simulink model "BMS_Protection_Logic"  (R2024a)
settings: Solver=VariableStepAuto  StartTime=0.0  StopTime=10.0  RelTol=1e-3
settings Model: Creator=gopin  LastModifiedBy=gopin

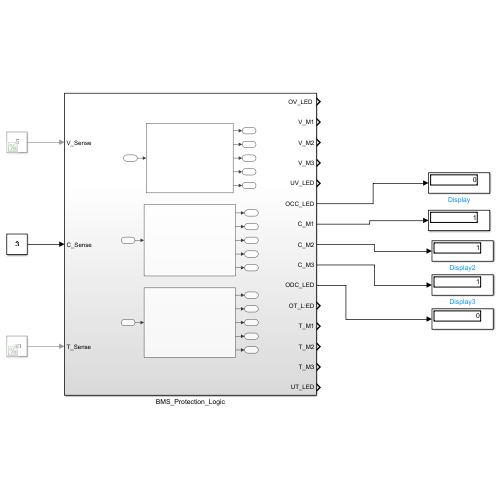
[thumbnail: Simulink's stored preview of the top-level diagram]
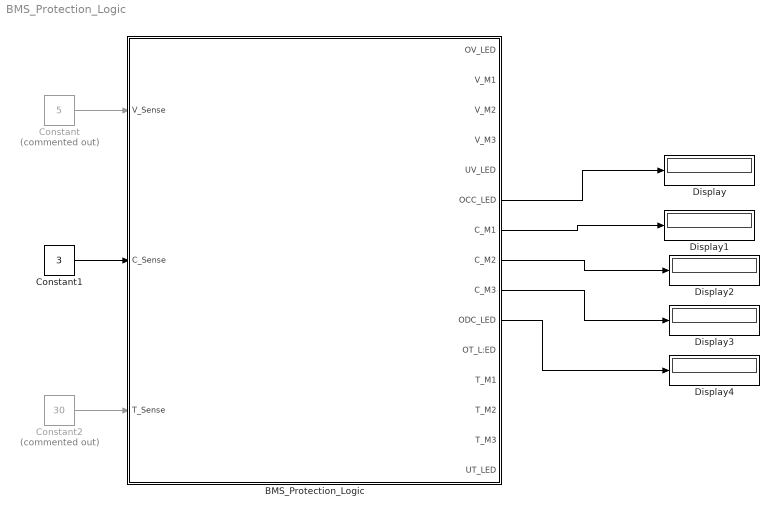
== system BMS_Protection_Logic ==
  BMS_Protection_Logic : Subsystem
  Constant : Constant  Commented=on  Value=5
  Constant1 : Constant  Value=3
  Constant2 : Constant  Commented=on  Value=30
  Display{,1..4} (5 alike) : Display
  wires:
  Constant/1 -> BMS_Protection_Logic/1(V_Sense)
  Constant1/1 -> BMS_Protection_Logic/2(C_Sense)
  Constant2/1 -> BMS_Protection_Logic/3(T_Sense)
  BMS_Protection_Logic/6(OCC_LED) -> Display/1
  BMS_Protection_Logic/7(C_M1) -> Display1/1
  BMS_Protection_Logic/8(C_M2) -> Display2/1
  BMS_Protection_Logic/9(C_M3) -> Display3/1
  BMS_Protection_Logic/10(ODC_LED) -> Display4/1

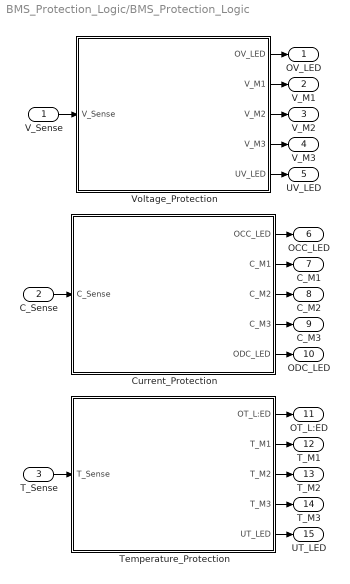
== system BMS_Protection_Logic/BMS_Protection_Logic ==
  V_Sense : Inport
  C_Sense : Inport  Port=2
  T_Sense : Inport  Port=3
  Current_Protection : Subsystem
  Temperature_Protection : Subsystem
  Voltage_Protection : Subsystem
  "OV_LED " : Outport
  V_M1 : Outport  Port=2
  V_M2 : Outport  Port=3
  V_M3 : Outport  Port=4
  UV_LED : Outport  Port=5
  OCC_LED : Outport  Port=6
  C_M1 : Outport  Port=7
  C_M2 : Outport  Port=8
  C_M3 : Outport  Port=9
  ODC_LED : Outport  Port=10
  OT_L:ED : Outport  Port=11
  T_M1 : Outport  Port=12
  T_M2 : Outport  Port=13
  T_M3 : Outport  Port=14
  UT_LED : Outport  Port=15
  wires:
  V_Sense/1 -> Voltage_Protection/1(V_Sense)
  Voltage_Protection/1("OV_LED ") -> "OV_LED "/1
  C_Sense/1 -> Current_Protection/1(C_Sense)
  Current_Protection/2(C_M1) -> C_M1/1
  Temperature_Protection/5(UT_LED) -> UT_LED/1
  Voltage_Protection/2(V_M1) -> V_M1/1
  Temperature_Protection/2(T_M1) -> T_M1/1
  Voltage_Protection/3(V_M2) -> V_M2/1
  Voltage_Protection/4(V_M3) -> V_M3/1
  Current_Protection/5(ODC_LED) -> ODC_LED/1
  Voltage_Protection/5(UV_LED) -> UV_LED/1
  Current_Protection/1(OCC_LED) -> OCC_LED/1
  Current_Protection/3(C_M2) -> C_M2/1
  Temperature_Protection/1(OT_L:ED) -> OT_L:ED/1
  T_Sense/1 -> Temperature_Protection/1(T_Sense)
  Current_Protection/4(C_M3) -> C_M3/1
  Temperature_Protection/3(T_M2) -> T_M2/1
  Temperature_Protection/4(T_M3) -> T_M3/1

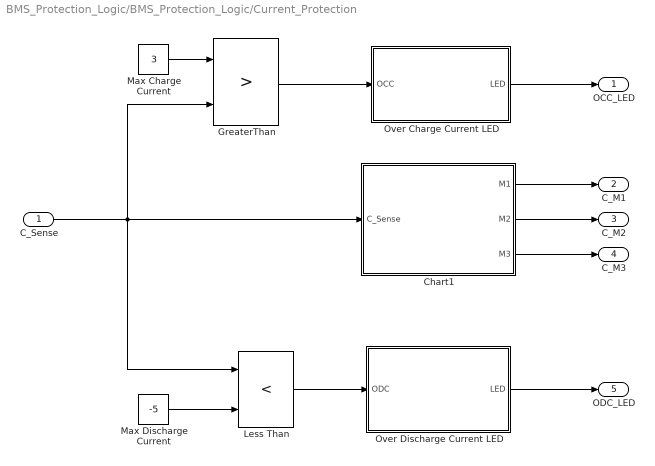
== system BMS_Protection_Logic/BMS_Protection_Logic/Current_Protection ==
  C_Sense : Inport
  Chart1 : Stateflow chart  TreatAsAtomicUnit=on
      settings: PortSchema="{\"entries\":[{\"content\":{\"sides\":[{\"content\":{\"connectorIds\":[\"In1\"]},\"type\":\"ConnectorPlacement.EquallySpacedRectSide\",\"uuid\":\"a6c9fd7f-8914-4577-a654-42bacf48963f\"},{\"content\":{\"connectorIds\":[\"Out2\",\"Out1\",\"Out3\"],\"side\":\"RIGHT\"},\"type\":\"ConnectorPlacement.EquallySpacedRectSide\",\"uuid\":\"5599986d-fed1-44ce-8dba-eb20f2a17f9b\"},{\"content\":{\"side\":\"TOP\"},\"type\":\"ConnectorPlacement.EquallySpacedRectSide\",\"uuid\":\"836751ae-26ce-4481-a9cd-daa336ec5618\"}]},\"type\":\"ConnectorPlacement.EquallySpacedConnector\",\"uuid\":\"966a675a-a05c-412b-8d9f-54425e62b931\"}],\"packageUris\":[\"http://schema.mathworks.com/mf0/Connector/R2020b\"],\"version\":\"1.0\"}"
  GreaterThan : RelationalOperator  Operator=>  OutDataTypeStr=boolean  RndMeth=Simplest  InputSameDT=off
  Less Than : RelationalOperator  Operator=<  OutDataTypeStr=boolean  RndMeth=Simplest  InputSameDT=off
  Max Charge Current : Constant  Value=3
  Max Discharge Current : Constant  Value=-5
  Over Charge Current LED : Stateflow chart  TreatAsAtomicUnit=on
  Over Discharge Current LED : Stateflow chart  TreatAsAtomicUnit=on
  OCC_LED : Outport
  C_M1 : Outport  Port=2
  C_M2 : Outport  Port=3
  C_M3 : Outport  Port=4
  ODC_LED : Outport  Port=5
  wires:
  Chart1/2(M1) -> C_M1/1
  Chart1/1(M2) -> C_M2/1
  Chart1/3(M3) -> C_M3/1
  C_Sense/1 -> Less Than/1, GreaterThan/2, Chart1/1(C_Sense)
  GreaterThan/1 -> Over Charge Current LED/1(OCC)
  Less Than/1 -> Over Discharge Current LED/1(ODC)
  Max Charge Current/1 -> GreaterThan/1
  Max Discharge Current/1 -> Less Than/2
  Over Discharge Current LED/1(LED) -> ODC_LED/1
  Over Charge Current LED/1(LED) -> OCC_LED/1

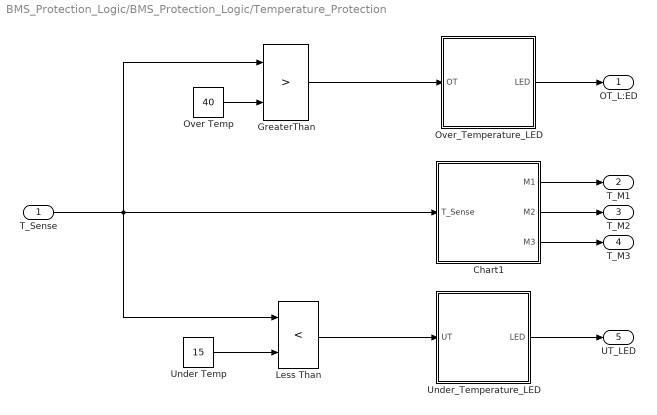
== system BMS_Protection_Logic/BMS_Protection_Logic/Temperature_Protection ==
  T_Sense : Inport
  Chart1 : Stateflow chart  TreatAsAtomicUnit=on
      settings: PortSchema="{\"entries\":[{\"content\":{\"sides\":[{\"content\":{\"connectorIds\":[\"In1\"]},\"type\":\"ConnectorPlacement.EquallySpacedRectSide\",\"uuid\":\"05ea740b-acd1-442a-a5fc-8d5534125df7\"},{\"content\":{\"connectorIds\":[\"Out1\",\"Out3\",\"Out2\"],\"side\":\"RIGHT\"},\"type\":\"ConnectorPlacement.EquallySpacedRectSide\",\"uuid\":\"8a7de145-2aa2-4311-b5d6-9482723dc71b\"},{\"content\":{\"side\":\"TOP\"},\"type\":\"ConnectorPlacement.EquallySpacedRectSide\",\"uuid\":\"63b1bd07-fd81-4427-8db4-3d8b6b536b2e\"}]},\"type\":\"ConnectorPlacement.EquallySpacedConnector\",\"uuid\":\"2e40ebd9-6121-4c1e-a234-5e0461cc6cd1\"}],\"packageUris\":[\"http://schema.mathworks.com/mf0/Connector/R2020b\"],\"version\":\"1.0\"}"
  GreaterThan : RelationalOperator  Operator=>  OutDataTypeStr=boolean  RndMeth=Simplest  InputSameDT=off
  Less Than : RelationalOperator  Operator=<  OutDataTypeStr=boolean  RndMeth=Simplest  InputSameDT=off
  Over Temp : Constant  Value=40
  Over_Temperature_LED : Stateflow chart  TreatAsAtomicUnit=on
  Under Temp : Constant  Value=15
  Under_Temperature_LED : Stateflow chart  TreatAsAtomicUnit=on
  OT_L:ED : Outport
  T_M1 : Outport  Port=2
  T_M2 : Outport  Port=3
  T_M3 : Outport  Port=4
  UT_LED : Outport  Port=5
  wires:
  GreaterThan/1 -> Over_Temperature_LED/1(OT)
  Less Than/1 -> Under_Temperature_LED/1(UT)
  Over Temp/1 -> GreaterThan/2
  Under Temp/1 -> Less Than/2
  T_Sense/1 -> GreaterThan/1, Chart1/1(T_Sense), Less Than/1
  Chart1/1(M1) -> T_M1/1
  Chart1/3(M2) -> T_M2/1
  Chart1/2(M3) -> T_M3/1
  Over_Temperature_LED/1(LED) -> OT_L:ED/1
  Under_Temperature_LED/1(LED) -> UT_LED/1

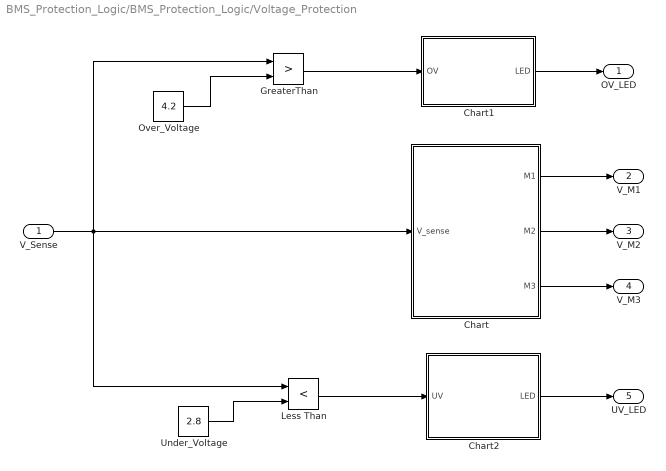
== system BMS_Protection_Logic/BMS_Protection_Logic/Voltage_Protection ==
  V_Sense : Inport
  Chart : Stateflow chart  TreatAsAtomicUnit=on
  Chart1 : Stateflow chart  TreatAsAtomicUnit=on
  Chart2 : Stateflow chart  TreatAsAtomicUnit=on
  GreaterThan : RelationalOperator  Operator=>  OutDataTypeStr=boolean  RndMeth=Simplest  InputSameDT=off
  Less Than : RelationalOperator  Operator=<  OutDataTypeStr=boolean  RndMeth=Simplest  InputSameDT=off
  Over_Voltage : Constant  Value=4.2
  Under_Voltage : Constant  Value=2.8
  "OV_LED " : Outport
  V_M1 : Outport  Port=2
  V_M2 : Outport  Port=3
  V_M3 : Outport  Port=4
  UV_LED : Outport  Port=5
  wires:
  Chart/1(M1) -> V_M1/1
  Chart/2(M2) -> V_M2/1
  Chart/3(M3) -> V_M3/1
  V_Sense/1 -> Less Than/1, GreaterThan/1, Chart/1(V_sense)
  Over_Voltage/1 -> GreaterThan/2
  Under_Voltage/1 -> Less Than/2
  Less Than/1 -> Chart2/1(UV)
  Chart1/1(LED) -> "OV_LED "/1
  Chart2/1(LED) -> UV_LED/1
  GreaterThan/1 -> Chart1/1(OV)

== stateflow chart BMS_Protection_Logic/Current_Protection/Over Discharge Current LED ==
  state LED_OFF
    en:
    LED=0;
    du:
    LED=0;
  state LED_ON
    en:
    LED=1;
  (default) -> LED_OFF
  LED_OFF -> LED_ON : [ODC==1]
  LED_ON -> LED_OFF : [ODC==0]
  data: ODC input; LED output

== stateflow chart BMS_Protection_Logic/Temperature_Protection/Over_Temperature_LED ==
  state LED_OFF
    en:
    LED=0;
    du:
    LED=0;
  state LED_ON
    en:
    LED=1;
  (default) -> LED_OFF
  LED_OFF -> LED_ON : [OT==1]
  LED_ON -> LED_OFF : [OT==0]
  data: LED output; OT input

== stateflow chart BMS_Protection_Logic/Temperature_Protection/Chart1 ==
  state OT_Cutoff
    en:
    M1=0;
    M2=0;
    M3=0;
  state Initial_Start
    en:
    M1=1;
    M2=1;
    M3=1;
  state UT_Cutoff
    en:
    M1=0;
    M2=0;
    M3=0;
  Initial_Start -> OT_Cutoff [order 1] : [T_Sense>40]
  (default) -> Initial_Start
  OT_Cutoff -> Initial_Start : [T_Sense<35 && after(10,sec)]
  Initial_Start -> UT_Cutoff [order 2] : [T_Sense<15]
  UT_Cutoff -> Initial_Start : [T_Sense>15 && after(10,sec)]
  data: M1 output; M3 output; M2 output; T_Sense input

== stateflow chart BMS_Protection_Logic/Temperature_Protection/Under_Temperature_LED ==
  state LED_OFF
    en:
    LED=0;
    du:
    LED=0;
  state LED_ON
    en:
    LED=1;
  (default) -> LED_OFF
  LED_OFF -> LED_ON : [UT==1]
  LED_ON -> LED_OFF : [UT==0]
  data: UT input; LED output

== stateflow chart BMS_Protection_Logic/Voltage_Protection/Chart1 ==
  state LED_ON
    en:
    LED=1;
  state LED_OFF
    en:
    LED=0;
    du:
    LED=0;
  (default) -> LED_OFF
  LED_OFF -> LED_ON : [OV==1]
  LED_ON -> LED_OFF : [OV==0]
  data: OV input; LED output

== stateflow chart BMS_Protection_Logic/Voltage_Protection/Chart2 ==
  state LED_ON
    en:
    LED=1;
  state LED_OFF
    en:
    LED=0;
    du:
    LED=0;
  (default) -> LED_OFF
  LED_OFF -> LED_ON : [UV==1]
  LED_ON -> LED_OFF : [UV==0]
  data: LED output; UV input

== stateflow chart BMS_Protection_Logic/Voltage_Protection/Chart ==
  state Charge
    en:
    M1=0;
    M2=0;
    M3=1;
  state Standby
    en:
    M1=1;
    M2=1;
    M3=1;
  state Setup
    en:
    M1=1;
    M3=1;
  state Setup1
    en:
    M1=1;
    M2=1;
  state DisCharge
    en:
    M1=0;
    M2=1;
    M3=0;
  Standby -> Charge [order 1] : [V_sense>4.15]
  (default) -> Standby
  Charge -> Standby [order 1] : [after(10,sec) && V_sense <4.0]
  Charge -> Setup [order 2] : [after(15,sec) && V_sense <=4.1]
  Setup -> Standby : [ V_sense >3 && V_sense <4.0]
  Setup1 -> Standby : [V_sense >3 && V_sense <4.0]
  DisCharge -> Standby [order 2] : [after(10,sec) && V_sense>=3.0]
  Standby -> DisCharge [order 2] : [V_sense<2.80]
  DisCharge -> Setup1 [order 1] : [after(15,sec) && V_sense>=2.85]
  data: V_sense input; M1 output; M2 output; M3 output

== stateflow chart BMS_Protection_Logic/Current_Protection/Over Charge Current LED ==
  state LED_OFF
    en:
    LED=0;
    du:
    LED=0;
  state LED_ON
    en:
    LED=1;
  (default) -> LED_OFF
  LED_OFF -> LED_ON : [OCC==1]
  LED_ON -> LED_OFF : [OCC==0]
  data: LED output; OCC input

== stateflow chart BMS_Protection_Logic/Current_Protection/Chart1 ==
  state Charge_Only
    en:
    M1=1;
    M2=1;
    M3=0;
  state Charge_Cutoff
    en:
    M1=0;
    M2=0;
  state Initial_Start
    en:
    M1=1;
    M2=1;
    M3=1;
  state Discharge_Only
    en:
    M1=1;
    M2=0;
    M3=1;
  state DisCharge_Cutoff
    en:
    M1=0;
    M3=0;
  Initial_Start -> Charge_Only [order 1] : [C_Sense < 2.5 && C_Sense>0.5]
  Charge_Only -> Charge_Cutoff [order 1] : [C_Sense >2.5]
  Charge_Cutoff -> Charge_Only [order 1] : [C_Sense < 2.5 && C_Sense>0.5 && after(10,sec)]
  Charge_Only -> Initial_Start [order 2] : [C_Sense < 0.5]
  (default) -> Initial_Start
  Charge_Cutoff -> Discharge_Only [order 2] : [C_Sense > -5  && C_Sense < -0.5]
  Charge_Only -> Discharge_Only [order 3] : [C_Sense < 2.5 && C_Sense>0.5]
  Discharge_Only -> Charge_Only [order 1] : [C_Sense > -5  && C_Sense < -0.5]
  DisCharge_Cutoff -> Charge_Only [order 2] : [C_Sense < 2.5 && C_Sense>0.5]
  Initial_Start -> Discharge_Only [order 2] : [C_Sense < -5 && C_Sense < -0.2]
  Discharge_Only -> Initial_Start [order 3] : [C_Sense > -0.2]
  Discharge_Only -> DisCharge_Cutoff [order 2] : [C_Sense < -5]
  DisCharge_Cutoff -> Discharge_Only [order 1] : [C_Sense > -5  && C_Sense < -0.5 && after(10,sec)]
  data: C_Sense input; M2 output; M1 output; M3 output
